simulink model "segway"  (R2020b)
settings: Solver=VariableStepAuto  StartTime=0.0  StopTime=7.0  RelTol=1e-3
undefined symbols (not defined in the file or in its folder): a21, a22, a31, a32, b2, b3, k1, k2, k3
settings Model: Creator=vital  LastModifiedBy=vital

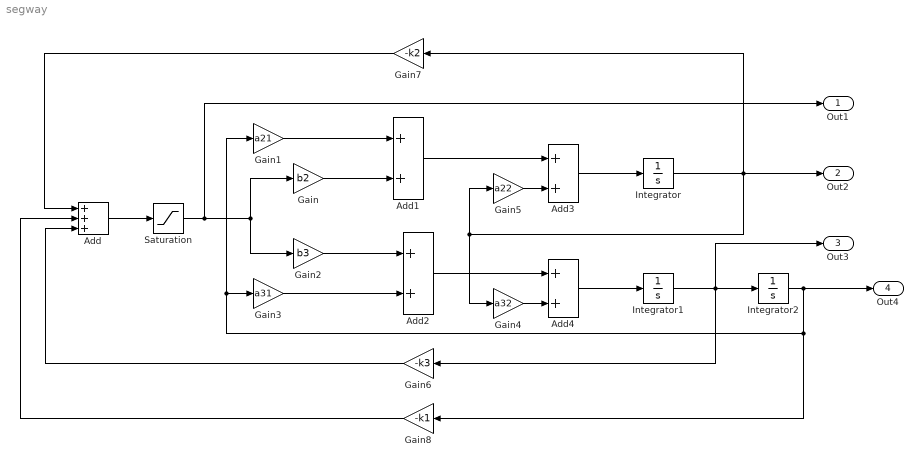
== system segway ==
  Add : Sum  Inputs=+++
  Add{1..4} (4 alike) : Sum
  Gain : Gain  Gain=b2
  Gain1 : Gain  Gain=a21
  Gain2 : Gain  Gain=b3
  Gain3 : Gain  Gain=a31
  Gain4 : Gain  Gain=a32
  Gain5 : Gain  Gain=a22
  Gain6 : Gain  Gain=-k3
  Gain7 : Gain  Gain=-k2
  Gain8 : Gain  Gain=-k1
  Integrator : Integrator
  Integrator1 : Integrator
  Integrator2 : Integrator  InitialCondition=pi/2
  Saturation : Saturate  UpperLimit=100  LowerLimit=-100
  Out1 : Outport  SignalName=Volt
  Out2 : Outport  Port=2  SignalName=dtheta
  Out3 : Outport  Port=3  SignalName=dpsi
  Out4 : Outport  Port=4  SignalName=psi
  wires:
  Add/1 -> Saturation/1
  Gain2/1 -> Add2/1
  Gain/1 -> Add1/2
  Gain1/1 -> Add1/1
  Saturation/1 -> Gain/1, Gain2/1, Out1/1
  Gain3/1 -> Add2/2
  Gain5/1 -> Add3/2
  Gain4/1 -> Add4/2
  Add1/1 -> Add3/1
  Add2/1 -> Add4/1
  Add3/1 -> Integrator/1
  Add4/1 -> Integrator1/1
  Integrator1/1 -> Gain6/1, Out3/1, Integrator2/1
  Integrator/1 -> Gain5/1, Gain4/1, Gain7/1, Out2/1
  Integrator2/1 -> Out4/1, Gain8/1, Gain1/1, Gain3/1
  Gain8/1 -> Add/2
  Gain6/1 -> Add/3
  Gain7/1 -> Add/1
